simulink model "ex2"  (Simulink 6.0)
settings: Solver=ode45  StartTime=0.0  StopTime=50.0  MaxStep=0.1  RelTol=1e-3
settings Model: LastModifiedBy=lxy

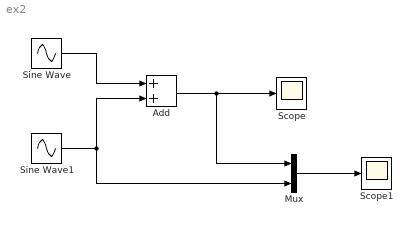
== system ex2 ==
  Add : Sum  OutScaling=2^-10
  Mux : Mux  Inputs=2
  Scope : Scope
  Scope1 : Scope
  Sine Wave : Sin  Amplitude=2  SampleTime=0
  Sine Wave1 : Sin  Frequency=2  Phase=pi/2  SampleTime=0
  wires:
  Sine Wave/1 -> Add/1
  Sine Wave1/1 -> Add/2, Mux/2
  Add/1 -> Scope/1, Mux/1
  Mux/1 -> Scope1/1
